simulink model "MPC Control"  (R2023b)
settings: Solver=FixedStepAuto  StartTime=0.0  StopTime=200  FixedStep=1e-2  RelTol=1e-3
InitFcn:
  | run('init.m');
undefined symbols (not defined in the file): CC, DiscIntNeverNeededParam, X0, Y0
libraries: simulink x2, mpclib x1
settings Model: Creator=Marvin  LastModifiedBy=刘宸鸣

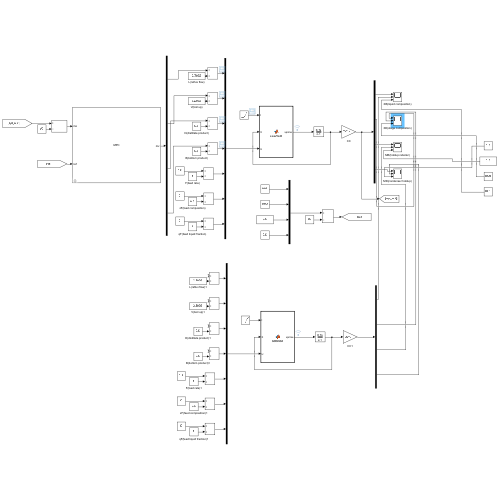
[thumbnail: Simulink's stored preview of the top-level diagram]
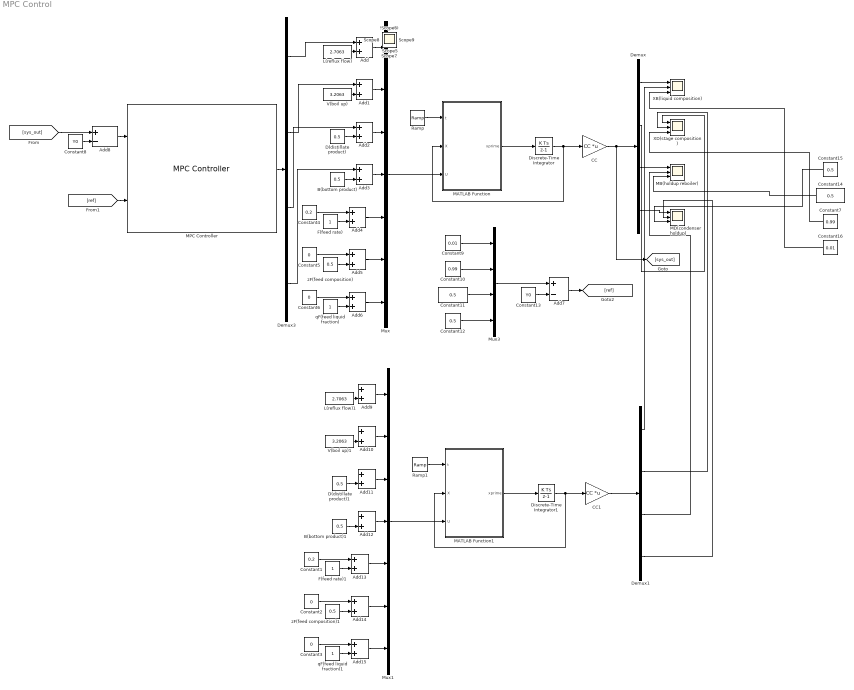
== system MPC Control ==
  Add{,1..6,9..15} (14 alike) : Sum
  Add7 : Sum  Inputs=+-
  Add8 : Sum  Inputs=+-
  B(bottom product) : Constant  Value=0.5
  B(bottom product)1 : Constant  Value=0.5
  CC : Gain  Gain=CC  Multiplication=Matrix(K*u)
  CC1 : Gain  Gain=CC  Multiplication=Matrix(K*u)
  Constant1 : Constant  Value=0.2
  Constant10 : Constant  Value=0.99
  Constant{11..12,14..15} (4 alike) : Constant  Value=0.5
  Constant13 : Constant  Value=Y0
  Constant16 : Constant  Value=0.01
  Constant{2..3,5..6} (4 alike) : Constant  Value=0
  Constant4 : Constant  Value=0.2
  Constant7 : Constant  Value=0.99
  Constant8 : Constant  Value=Y0
  Constant9 : Constant  Value=0.01
  D(distillate product) : Constant  Value=0.5
  D(distillate product)1 : Constant  Value=0.5
  Demux : Demux
  Demux1 : Demux
  Demux3 : Demux
  Discrete-Time Integrator : DiscreteIntegrator  InitialCondition=X0  SampleTime=-1  ICPrevOutput=DiscIntNeverNeededParam  ICPrevScaledInput=DiscIntNeverNeededParam
  Discrete-Time Integrator1 : DiscreteIntegrator  InitialCondition=X0  SampleTime=-1  ICPrevOutput=DiscIntNeverNeededParam  ICPrevScaledInput=DiscIntNeverNeededParam
  F(feed rate) : Constant
  F(feed rate)1 : Constant
  L(reflux flow) : Constant  Value=2.7063
  L(reflux flow)1 : Constant  Value=2.7063
  MATLAB Function : MATLAB Function  TreatAsAtomicUnit=on
  MATLAB Function1 : MATLAB Function  TreatAsAtomicUnit=on
  MB(holdup reboiler) : Scope  NumInputPorts=3
  MD(condenser holdup) : Scope  NumInputPorts=3
  MPC Controller : mpclib/MPC Controller  SCDEnableBlockLinearizationSpecification=on  mpcobj=mpc_controller  x0=x0  is_multiple=0  enable_value=0  return_u0=off  updateMPCinCallerWorkspace=on  md_inport=off  mv_inport=off  uref_inport=off  return_cost=off  return_mvseq=off  return_qpstatus=off  return_xseq=off  return_state=off  return_ovseq=off  state_inport=off  umin_inport=off  umax_inport=off  ymin_inport=off  ymax_inport=off  cc_inport=off  ywt_inport=off  uwt_inport=off  duwt_inport=off  rhoeps_inport=off  pm_inport=off  MaximumP=10  HorizonChoice=FixedHorizon  n_ts=0.01  n_p=300  n_mv=4  n_md=0  n_ud=0  n_mo=4  n_uo=0  BlockDataType=double  SampleTimeInherited=off  switch_inport=off
  Mux : Mux  Inputs=7
  Mux1 : Mux  Inputs=7
  Mux3 : Mux
  Ramp : simulink/Sources/Ramp  slope=1  start=0  InitialOutput=0
  Ramp1 : simulink/Sources/Ramp  slope=1  start=0  InitialOutput=0
  V(boil up) : Constant  Value=3.2063
  V(boil up)1 : Constant  Value=3.2063
  XB(liquid composition) : Scope  NumInputPorts=3
  XD(stage composition) : Scope  NumInputPorts=3
  qF(feed liquid fraction) : Constant
  qF(feed liquid fraction)1 : Constant
  zF(feed composition) : Constant  Value=0.5
  zF(feed composition)1 : Constant  Value=0.5
  Scope{,1..10} (11 alike) : Scope
  wires:
  Ramp/1 -> MATLAB Function/1(t)
  MATLAB Function/1(xprime) -> Discrete-Time Integrator/1
  Discrete-Time Integrator/1 -> MATLAB Function/2(X), CC/1
  CC/1 -> [sys_out], Demux/1
  Demux/3 -> MB(holdup reboiler)/1
  Demux/2 -> XD(stage composition)/1
  Add1/1 -> Mux/2
  Add2/1 -> Mux/3
  Add3/1 -> Mux/4
  Add4/1 -> Mux/5
  F(feed rate)/1 -> Add4/2
  Constant4/1 -> Add4/1
  Add5/1 -> Mux/6
  zF(feed composition)/1 -> Add5/2
  Constant5/1 -> Add5/1
  Add6/1 -> Mux/7
  qF(feed liquid fraction)/1 -> Add6/2
  Constant6/1 -> Add6/1
  L(reflux flow)/1 -> Add/2
  V(boil up)/1 -> Add1/2
  D(distillate product)/1 -> Add2/2
  B(bottom product)/1 -> Add3/2
  Demux/1 -> XB(liquid composition)/1
  Demux/4 -> MD(condenser holdup)/1
  Add/1 -> Mux/1
  Demux3/1 -> Add/1
  Mux/1 -> MATLAB Function/3(U)
  Demux3/2 -> Add1/1
  Demux3/3 -> Add2/1
  [sys_out] -> Add8/1
  [ref] -> MPC Controller/2
  MPC Controller/1 -> Demux3/1
  Add8/1 -> MPC Controller/1
  Constant8/1 -> Add8/2
  Constant9/1 -> Mux3/1
  Constant10/1 -> Mux3/2
  Constant11/1 -> Mux3/3
  Constant12/1 -> Mux3/4
  Mux3/1 -> Add7/1
  Add7/1 -> [ref]
  Constant13/1 -> Add7/2
  Demux3/4 -> Add3/1
  Add9/1 -> Mux1/1
  Mux1/1 -> MATLAB Function1/3(U)
  V(boil up)1/1 -> Add10/2
  Add12/1 -> Mux1/4
  L(reflux flow)1/1 -> Add9/2
  Discrete-Time Integrator1/1 -> MATLAB Function1/2(X), CC1/1
  B(bottom product)1/1 -> Add12/2
  CC1/1 -> Demux1/1
  D(distillate product)1/1 -> Add11/2
  Add10/1 -> Mux1/2
  Ramp1/1 -> MATLAB Function1/1(t)
  Add11/1 -> Mux1/3
  MATLAB Function1/1(xprime) -> Discrete-Time Integrator1/1
  F(feed rate)1/1 -> Add13/2
  zF(feed composition)1/1 -> Add14/2
  Constant3/1 -> Add15/1
  Constant2/1 -> Add14/1
  Constant1/1 -> Add13/1
  Add13/1 -> Mux1/5
  Add14/1 -> Mux1/6
  qF(feed liquid fraction)1/1 -> Add15/2
  Add15/1 -> Mux1/7
  Demux1/1 -> XB(liquid composition)/2
  Demux1/2 -> XD(stage composition)/2
  Demux1/3 -> MB(holdup reboiler)/2
  Demux1/4 -> MD(condenser holdup)/2
  Constant16/1 -> XB(liquid composition)/3
  Constant7/1 -> XD(stage composition)/3
  Constant14/1 -> MB(holdup reboiler)/3
  Constant15/1 -> MD(condenser holdup)/3

== matlab function MPC Control/MATLAB Function ==
  data: t input; xprime output; X input; U input
function xprime=colamod(t,X,U)
%
% colamod - This is a nonlinear model of a distillation column with
%           NT-1 theoretical stages including a reboiler (stage 1) plus a
%           total condenser ("stage" NT). The liquid flow dynamics are
%           modelled by a simple linear relationship.
%           Model assumptions: Two components (binary separation); constant
%           relative volatility; no vapor holdup; one feed and two products;
%           constant molar flows (same vapor flow on all stages);
%           total condenser
%
%           The model is based on column A in Skogestad and Postlethwaite
%           (1996). The model has 82 states.
%
% Inputs:    t    - time in [min].
%            X    - State, the first 41 states are compositions of light
%                   component A with reboiler/bottom stage as X(1) and
%                   condenser as X(41). State X(42)is holdup in reboiler/
%                   bottom stage and X(82) is hold-up in condenser.
%            U(1) - reflux L,
%            U(2) - boilup V,
%            U(3) - top or distillate product flow D,
%            U(4) - bottom product flow B,
%            U(5) - feed rate F,
%            U(6) - feed composition, zF.
%            U(7) - feed liquid fraction, qF.
%
% Outputs:   xprime - vector with time derivative of all the states
%%%%%%%%%%%%%%%%%%%%%%%%%%%%%%%%%%%%%%%%%%%%%%%%%%%%%%%%%

%------------------------------------------------------------
% The following data need to be changed for a new column.
% These data are for "colmn A".
% Number of stages (including reboiler and total condenser:
NT=41;
% Location of feed stage (stages are counted from the bottom):
NF=21;
% Relative volatility
alpha=1.5;
% Nominal liquid holdups
M0 = zeros(1,NT);
M0(1)=0.5;      	% Nominal reboiler holdup (kmol)
i=2:NT-1; M0(i)=0.5*ones(1,NT-2);% Nominal stage (tray) holdups (kmol)
M0(NT)=0.5;      	% Nominal condenser holdup (kmol)
% Data for linearized liquid flow dynamics (does not apply to reboiler and condenser):
taul=0.063;     	% time constant for liquid dynamics (min)
F0=1;	 	% Nominal feed rate (kmol/min)
qF0 = 1; 		% Nominal fraction of liquid in feed
L0=2.70629;     	% Nominal reflux flow (from steady-state data)
L0b=L0 + qF0*F0;	% Nominal liquid flow below feed (kmol/min)
lambda=0;		% Effect of vapor flow on liquid flow ("K2-effect")
V0=3.20629;V0t=V0+(1-qF0)*F0;% Nominal vapor flows - only needed if lambda is nonzero
% End data which need to be changed
%------------------------------------------------------------

% Splitting the states
x=X(1:NT)';                          % Liquid composition from btm to top
M=X(NT+1:2*NT)';                     % Liquid hold up from btm to top

% Inputs and disturbances
LT = U(1);                            % Reflux
VB = U(2);                            % Boilup
D  = U(3);                            % Distillate
B  = U(4);                            % Bottoms

F  = U(5);                            % Feedrate
zF = U(6);                            % Feed composition
qF = U(7);                            % Feed liquid fraction

% THE MODEL

y = zeros(1,NT);
% Vapor-liquid equilibria
for i=1:1:NT-1
    y(i)=alpha*x(i)./(1+(alpha-1)*x(i));
end

% Vapor Flows assuming constant molar flows

V = VB*ones(1,NT-1);

for i=NF:1:NT-1
    V(i)=V(i) + (1-qF)*F;
end

% Liquid flows assuming linearized tray hydraulics with time constant taul
% Also includes coefficient lambda for effect of vapor flow ("K2-effect").
L = zeros(1,NT);
for i=2:1:NF
    L(i) = L0b + (M(i)-M0(i))./taul + lambda.*(V(i-1)-V0);
end

for i=NF+1:1:NT-1
L(i) = L0  + (M(i)-M0(i))./taul + lambda.*(V(i-1)-V0t);
end



L(NT)=LT;

% Time derivatives from  material balances for
% 1) total holdup and 2) component holdup

% Column
dMdt = zeros(1,NT);
dMxdt = zeros(1,NT);
for i=2:1:NT-1
dMdt(i) = L(i+1)         - L(i)       + V(i-1)         - V(i);
dMxdt(i)= L(i+1).*x(i+1) - L(i).*x(i) + V(i-1).*y(i-1) - V(i).*y(i);
end
% Correction for feed at the feed stage
% The feed is assumed to be mixed into the feed stage
dMdt(NF) = dMdt(NF)  + F;
dMxdt(NF)= dMxdt(NF) + F*zF;

% Reboiler (assumed to be an equilibrium stage)
dMdt(1) = L(2)      - V(1)      - B;
dMxdt(1)= L(2)*x(2) - V(1)*y(1) - B*x(1);

% Total condenser (no equilibrium stage)
dMdt(NT) = V(NT-1)         - LT       - D;
dMxdt(NT)= V(NT-1)*y(NT-1) - LT*x(NT) - D*x(NT);

% Compute the derivative for the mole fractions from d(Mx) = x dM + M dx
dxdt = zeros(1,NT);
for i=1:1:NT
dxdt(i) = (dMxdt(i) - x(i).*dMdt(i) )./M(i);
end

% Output
xprime=[dxdt';dMdt'];

end

== matlab function MPC Control/MATLAB Function1 ==
  data: t input; xprime output; X input; U input
function xprime=colamod(t,X,U)
%
% colamod - This is a nonlinear model of a distillation column with
%           NT-1 theoretical stages including a reboiler (stage 1) plus a
%           total condenser ("stage" NT). The liquid flow dynamics are
%           modelled by a simple linear relationship.
%           Model assumptions: Two components (binary separation); constant
%           relative volatility; no vapor holdup; one feed and two products;
%           constant molar flows (same vapor flow on all stages);
%           total condenser
%
%           The model is based on column A in Skogestad and Postlethwaite
%           (1996). The model has 82 states.
%
% Inputs:    t    - time in [min].
%            X    - State, the first 41 states are compositions of light
%                   component A with reboiler/bottom stage as X(1) and
%                   condenser as X(41). State X(42)is holdup in reboiler/
%                   bottom stage and X(82) is hold-up in condenser.
%            U(1) - reflux L,
%            U(2) - boilup V,
%            U(3) - top or distillate product flow D,
%            U(4) - bottom product flow B,
%            U(5) - feed rate F,
%            U(6) - feed composition, zF.
%            U(7) - feed liquid fraction, qF.
%
% Outputs:   xprime - vector with time derivative of all the states
%%%%%%%%%%%%%%%%%%%%%%%%%%%%%%%%%%%%%%%%%%%%%%%%%%%%%%%%%

%------------------------------------------------------------
% The following data need to be changed for a new column.
% These data are for "colmn A".
% Number of stages (including reboiler and total condenser:
NT=41;
% Location of feed stage (stages are counted from the bottom):
NF=21;
% Relative volatility
alpha=1.5;
% Nominal liquid holdups
M0 = zeros(1,NT);
M0(1)=0.5;      	% Nominal reboiler holdup (kmol)
i=2:NT-1; M0(i)=0.5*ones(1,NT-2);% Nominal stage (tray) holdups (kmol)
M0(NT)=0.5;      	% Nominal condenser holdup (kmol)
% Data for linearized liquid flow dynamics (does not apply to reboiler and condenser):
taul=0.063;     	% time constant for liquid dynamics (min)
F0=1;	 	% Nominal feed rate (kmol/min)
qF0 = 1; 		% Nominal fraction of liquid in feed
L0=2.70629;     	% Nominal reflux flow (from steady-state data)
L0b=L0 + qF0*F0;	% Nominal liquid flow below feed (kmol/min)
lambda=0;		% Effect of vapor flow on liquid flow ("K2-effect")
V0=3.20629;V0t=V0+(1-qF0)*F0;% Nominal vapor flows - only needed if lambda is nonzero
% End data which need to be changed
%------------------------------------------------------------

% Splitting the states
x=X(1:NT)';                          % Liquid composition from btm to top
M=X(NT+1:2*NT)';                     % Liquid hold up from btm to top

% Inputs and disturbances
LT = U(1);                            % Reflux
VB = U(2);                            % Boilup
D  = U(3);                            % Distillate
B  = U(4);                            % Bottoms

F  = U(5);                            % Feedrate
zF = U(6);                            % Feed composition
qF = U(7);                            % Feed liquid fraction

% THE MODEL

y = zeros(1,NT);
% Vapor-liquid equilibria
for i=1:1:NT-1
    y(i)=alpha*x(i)./(1+(alpha-1)*x(i));
end

% Vapor Flows assuming constant molar flows

V = VB*ones(1,NT-1);

for i=NF:1:NT-1
    V(i)=V(i) + (1-qF)*F;
end

% Liquid flows assuming linearized tray hydraulics with time constant taul
% Also includes coefficient lambda for effect of vapor flow ("K2-effect").
L = zeros(1,NT);
for i=2:1:NF
    L(i) = L0b + (M(i)-M0(i))./taul + lambda.*(V(i-1)-V0);
end

for i=NF+1:1:NT-1
L(i) = L0  + (M(i)-M0(i))./taul + lambda.*(V(i-1)-V0t);
end



L(NT)=LT;

% Time derivatives from  material balances for
% 1) total holdup and 2) component holdup

% Column
dMdt = zeros(1,NT);
dMxdt = zeros(1,NT);
for i=2:1:NT-1
dMdt(i) = L(i+1)         - L(i)       + V(i-1)         - V(i);
dMxdt(i)= L(i+1).*x(i+1) - L(i).*x(i) + V(i-1).*y(i-1) - V(i).*y(i);
end
% Correction for feed at the feed stage
% The feed is assumed to be mixed into the feed stage
dMdt(NF) = dMdt(NF)  + F;
dMxdt(NF)= dMxdt(NF) + F*zF;

% Reboiler (assumed to be an equilibrium stage)
dMdt(1) = L(2)      - V(1)      - B;
dMxdt(1)= L(2)*x(2) - V(1)*y(1) - B*x(1);

% Total condenser (no equilibrium stage)
dMdt(NT) = V(NT-1)         - LT       - D;
dMxdt(NT)= V(NT-1)*y(NT-1) - LT*x(NT) - D*x(NT);

% Compute the derivative for the mole fractions from d(Mx) = x dM + M dx
dxdt = zeros(1,NT);
for i=1:1:NT
dxdt(i) = (dMxdt(i) - x(i).*dMdt(i) )./M(i);
end

% Output
xprime=[dxdt';dMdt'];

end
